simulink subsystem "s0502_Bad_Energy"  (R2019b)
settings: Solver=VariableStepAuto  StartTime=0.0  StopTime=10.0  RelTol=1e-3
model mask{K_th=0, K_th_dot=0, K_al=0, K_al_dot=0}
undefined symbols (not defined in the file): __PRM__SERIALIZED__DATA__, PARAMS, SubsystemReferenceBlock
settings Model: Creator=francescoceresetti  LastModifiedBy=alessandro

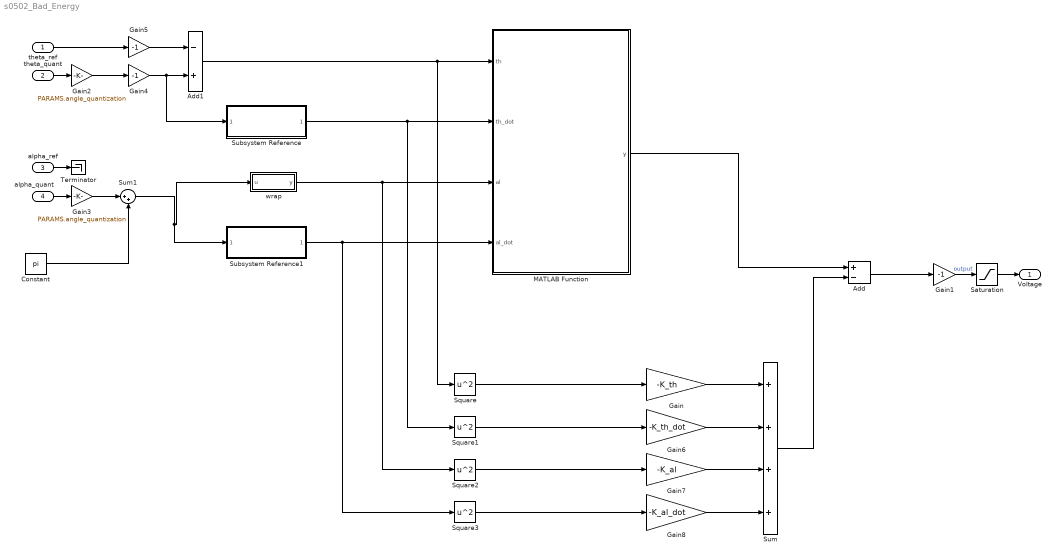
== system s0502_Bad_Energy ==
  theta_ref : Inport
  theta_quant : Inport  Port=2
  alpha_ref : Inport  Port=3
  alpha_quant : Inport  Port=4
  Add : Sum  Inputs=+-
  Add1 : Sum  Inputs=-+
  Constant : Constant  Value=pi
  Gain : Gain  Gain=-K_th
  Gain1 : Gain  Gain=-1
  Gain2 : Gain  Gain=PARAMS.angle_quantization
  Gain3 : Gain  Gain=PARAMS.angle_quantization
  Gain4 : Gain  Gain=-1
  Gain5 : Gain  Gain=-1
  Gain6 : Gain  Gain=-K_th_dot
  Gain7 : Gain  Gain=-K_al
  Gain8 : Gain  Gain=-K_al_dot
  MATLAB Function : MATLAB Function  TreatAsAtomicUnit=on
  Saturation : Saturate  UpperLimit=PARAMS.V_sat  LowerLimit=-PARAMS.V_sat
  Square{,1..3} (4 alike) : Math  Operator=square  SignedPower=off  SaturateOnIntegerOverflow=on
  Subsystem Reference : Subsystem  BlockKeywords=__PRM__SERIALIZED__DATA__:SubsystemReferenceBlock  ReferencedSubsystem=Filtered_Derivative  num=num_der_filter  den=den_der_filter
  Subsystem Reference1 : Subsystem  BlockKeywords=__PRM__SERIALIZED__DATA__:SubsystemReferenceBlock  ReferencedSubsystem=Filtered_Derivative  num=num_der_filter  den=den_der_filter
  Sum : Sum  Inputs=++++
  Sum1 : Sum  Inputs=|++
  Terminator : Terminator
  wrap : MATLAB Function  TreatAsAtomicUnit=on
  Voltage : Outport
  wires:
  alpha_quant/1 -> Gain3/1
  Add1/1 -> Square/1, MATLAB Function/1(th)
  theta_quant/1 -> Gain2/1
  Subsystem Reference1/1 -> MATLAB Function/4(al_dot), Square3/1
  Subsystem Reference/1 -> MATLAB Function/2(th_dot), Square1/1
  Gain3/1 -> Sum1/1
  wrap/1(y) -> MATLAB Function/3(al), Square2/1
  Saturation/1 -> Voltage/1
  Gain4/1 -> Add1/2, Subsystem Reference/1
  Gain5/1 -> Add1/1
  theta_ref/1 -> Gain5/1
  Gain2/1 -> Gain4/1
  Gain1/1 -> Saturation/1  "output"
  alpha_ref/1 -> Terminator/1
  Add/1 -> Gain1/1
  MATLAB Function/1(y) -> Add/1
  Square/1 -> Gain/1
  Gain/1 -> Sum/1
  Square1/1 -> Gain6/1
  Gain6/1 -> Sum/2
  Square2/1 -> Gain7/1
  Gain7/1 -> Sum/3
  Square3/1 -> Gain8/1
  Gain8/1 -> Sum/4
  Sum/1 -> Add/2
  Sum1/1 -> wrap/1(u), Subsystem Reference1/1
  Constant/1 -> Sum1/2

== matlab function s0502_Bad_Energy/MATLAB Function ==
  data: th input; y output; th_dot input; al input; al_dot input; PARAMS parameter
function y = fcn(th, th_dot, al, al_dot, PARAMS)
    T_eq = (39.6456*al_dot + 1.23139*th_dot^3*sin(al) - 12.6196*al*al_dot - 15.5921*al_dot*cos(2.0*al) + 103.345*th*th_dot - 103.345*th_0*th_dot - 0.302991*al_dot^2*cos(2.0*al) + 2.78626*al_dot^3*sin(2.0*al) + 2.14428*al_dot^2 + 1.23139*th_dot^3*sin(3.0*al) + 16.0519*th_dot^2 - 3.34917*al_dot*th_dot^2*sin(2.0*al) + 0.544219*al_dot*th_dot^2*sin(4.0*al) - 2.46279*al_dot^2*th_dot*sin(3.0*al) - 7.38837*al_dot^2*th_dot*sin(al) + 4.96313*al*al_dot*cos(2.0*al) - 32.7795*g*th_dot*sin(2.0*al) - 14.487*al_dot*g*sin(3.0*al) - 116.919*al_dot*th*cos(al) + 116.919*al_dot*th_0*cos(al) - 18.8457*al_dot*th_dot*cos(al) + 219.537*al_dot*g*sin(al))/(46657.0*th_dot - 52785.0*al_dot*cos(al));
    
    V = PARAMS.Rm*T_eq/PARAMS.ki + PARAMS.kv*th_dot;
    
y = V;

== matlab function s0502_Bad_Energy/wrap ==
  data: u input; y output
function y = wrap(u)
stop_condition = false;
y = u;
while ~stop_condition
    if y > pi
        y = y - 2*pi;
    elseif y < -pi
        y = y + 2*pi;
    else
        stop_condition = true;
    end
end
